simulink model "EcoSIM3_P2_C2"  (R2014b)
settings: Solver=ode1  SolverMode=SingleTasking  StartTime=0.0  StopTime=inf  FixedStep=0.01  RelTol=1e-3
PostLoadFcn:
  | %, if any(exist('dsrtsu_mdlpostloadfcn', 'file') == [2, 3, 6]), try dsrtsu_mdlpostloadfcn('Execute', bdroot); catch fprintf('Error in PostLoadFcn (dsrtsu_mdlpostloadfcn) for model "%s":\n %s\n', bdroot, lasterr); end, end,
InitFcn:
  | tic
  | %Startup_EcoSIM
values from neighbouring files (symbols this model uses):
  EngPwr = [0 5	10	15	20	25	30	35	40	45	50	55	60	65	70	75	80	85	90	95	100	105	110	115]    [Series_Maps.m]
  EngSpd = [0 477.4645 954.929 1909.858 2864.787 3819.716 4774.645 5729.574 6684.503]    [Series_Maps.m]
  EngTrq = [0	0	0	0	0	0	0	0	0	0	0	0	0	0	0	0	0	0	0	0	0	0	0	0 ... (first row only)    [Series_Maps.m]
  Power = [0 5 10 15 20 25 30]    [Series_Maps.m]
  Torque = [-50,-40,-30,-25,-20,-15,-10,-8,-6,-4,-2,0]    [Series_Maps.m]
undefined symbols (not defined in the file or in its folder): canChannel, Controls, DriveCycles, Driver, EM_EFF_MAP, EM_PwrLoss_MAP, Glbl, Plants, Veh_Dynamics
libraries: canmsglib x100, canlib x87, fl_lib x78, simulink x59, nesl_utility x40, sdl_lib x17, dspsigops x5, dspswit3 x3, dspstat3 x2, commnoisgen2 x1, dspfdesign x1
(part 1 of 15)
settings Model: DSRTSU_INTERNAL_RTI_VER=450  DSRTSU_INTERNAL_RTI_TYPE=rti1006  RTICANMMDATA=struct('GeneralSetupData',struct('modelroot','C:\Users\EcoCAR_HIL\Documents\Khanna\EcoSIM3_P1_0_PHEV_dynamic_RTI','generalsettings',struct('filesettings',struct('destfolder',struct('Name','RTICANMM_FILES','Check',1),'buildfolder',struct('Name','.','Check',1),'AbsDestfolder',struct('Name','C:\Users\EcoCAR_HIL\Documents\Khanna\EcoSIM3_P1_0_PHEV_dynamic_RTI\RTICANMM_FILES'),'AbsBuildfolder',struct('Name','C:\Users\EcoCAR_HIL\Documents\Khanna\EcoSIM3_P1_0_PHEV_dynamic_RTI'))),'options',struct('addpaths',1,'rmpaths',1,'addtrcexclusion',logical(1),'cannavigator',struct('checkmonitoring',0),'show_usrtrc',0,'use_usrtrc',0),'advanced',struct('options',[1 1 1 1 1 1 1 1 1 1 1 1 1 1 1 1 1 1 1 1 1 1 1 1 1 1 1 1 1 1 1 1 1 1 1 1 1 1 1 1 1 1 1 1 1 1 1 1 1 1 1 1 1 1 1 1 1 1 1 1 1 1 1 1 1 1 1 1 1 1 1 1 1 1 1 1 1 1 1 1 1 1 1 1 1 1 1 1 1 1 1 1 1 1 1 1 1 1 1 1]),'MPSetup',{{}},'modelname','EcoSIM3_P1_0_PHEV_2014b_with_inertia','block','EcoSIM3_P1_0_PHEV_2014b_with_inertia'))  DSRTSU_INTERNAL_RTIFPGA=40  Creator=Arjun  LastModifiedBy=EcoCAR_HIL
settings ConfigSet: Description=This configuration is meant for HIL simulations. During HIL simulations, the model should use dSPACE's rti1006 to generate code.
settings DataIOCC: InspectSignalLogs=on
settings OptimizationCC: BlockReduction=off
settings DebuggingCC: UnderspecifiedInitializationDetection=Classic  MergeDetectMultiDrivingBlocksExec=none  MultiTaskCondExecSysMsg=warning
settings HardwareCC: ProdIntDivRoundTo=Zero  ProdEndianess=LittleEndian  ProdHWDeviceType=Generic->Custom  TargetIntDivRoundTo=Zero  TargetEndianess=LittleEndian  TargetHWDeviceType=Generic->Custom
settings RTWCC: SystemTargetFile=rti1006.tlc  MakeCommand=make_rti  TemplateMakefile=rti1006.tmf  Description=dSPACE DS1006 Hardware Platform  ProcessScript=rti1006_make_rtw_hook
settings STFCustomTargetCC: ParMdlRefBuildCompliant=on  GeneratePreprocessorConditionals=Disable all  SystemTargetFile=rti1006.tlc
settings GRTTargetCC: CompOptLevelCompliant=off  ConcurrentExecutionCompliant=off  CombineOutputUpdateFcns=off  MatFileLogging=off  CPPClassGenCompliant=off  GRTInterface=on  ExtModeMexFile=noextcomm
settings SimscapeCC: SelectedTab=Simscape

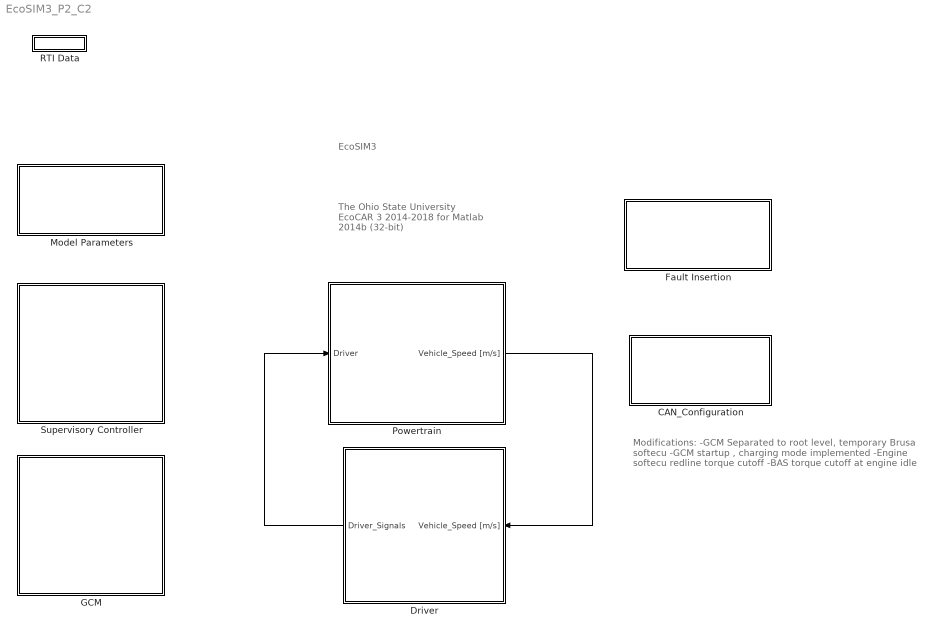
== system EcoSIM3_P2_C2 ==
  note: Modifications:
      | -GCM Separated to root level, temporary Brusa softecu
      | -GCM startup , charging mode implemented
      | -Engine softecu redline torque cutoff
      | -BAS torque cutoff at engine idle
  note: The Ohio State University
      | EcoCAR 3 2014-2018
      | for Matlab 2014b (32-bit)
  note: EcoSIM3
  CAN_Configuration : Subsystem  Variant=on  VariantControl=Sim_type == 1
  Driver : Subsystem
      mask Display: image(imread('images/BRUTUS.png'))
  Fault Insertion : Subsystem
  GCM : Subsystem  SystemSampleTime=0.001  VariantControl=Variant1
      settings: MinAlgLoopOccurrences=on
      mask Display: image(imread('images/GCM.jpg'))
  Model Parameters : Subsystem  mask{DRIV_cycle=US06 - City portion, Grade=0, Init_SOC=50}
      mask prompts: DRIV_cycle "Drive Cycle"; Grade "Grade [%]"; Init_SOC "Initial SOC [%]"
      mask help: Model Parameters Available for Modification
      mask TypeOptions DRIV_cycle: FUDS | FHDS | US06 | UDDS - 505 portion | US06 - City portion | US06 - Highway portion | Gradeability Test | Acceleration Test | Demo Cycle
      mask Display: disp('Simulation\nParameters')
  Powertrain : Subsystem
      mask Display: image(imread('images/OSU_EC3_Powertrain.png'))
  RTI Data : Subsystem  Tag=struct('RTIDataServer',struct('RTIDataServerVs','2','RTIModelDescription','struct(''main'',''EcoSIM3_P2_C2'',''sub'','''',''isMp'',0)'))  LoadFcn="if exist('rtidc'), try,  rtidc('DataHostBlockClbLoad', gcbh); catch, disp(['Warning: ''LoadFcn'' for RTI Data block failed: ' lasterr]); end, end,"  mask(RTI_DATA_HOST){}
      mask help:
      | RTI Data Block.
      | This block is used by RTI to store internal model-dependent data.
      | Please keep this block on the root level of the model. Deleting this block will result in data loss.
      |
      | NEVER DELETE OR COPY THIS BLOCK!
      settings: CopyFcn="if exist('rtidc'), try,  rtidc('DataHostBlockClbCopy', gcbh); catch, disp(['Warning: ''CopyFcn'' for RTI Data block failed: ' lasterr]); end, end,"  DeleteFcn="if exist('rtidc'), try,  rtidc('DataHostBlockClbDelete', gcbh); catch, disp(['Warning: ''DeleteFcn'' for RTI Data block failed: ' lasterr]); end, end,"  ModelCloseFcn="if exist('rtidc'), try,  rtidc('DataHostBlockClbModelClose', gcbh); catch, disp(['Warning: ''ModelCloseFcn'' for RTI Data block failed: ' lasterr]); end, end,"  PreSaveFcn="if exist('rtidc'), try,  rtidc('DataHostBlockClbPreSave', gcbh); catch, disp(['Warning: ''PreSaveFcn'' for RTI Data block failed: ' lasterr]); end, end,"  PostSaveFcn="if exist('rtidc'), try,  rtidc('DataHostBlockClbPostSave', gcbh); catch, disp(['Warning: ''PostSaveFcn'' for RTI Data block failed: ' lasterr]); end, end,"  NameChangeFcn="if exist('rtidc'), try,  rtidc('DataHostBlockClbNameChange', gcbh); catch, disp(['Warning: ''NameChangeFcn'' for RTI Data block failed: ' lasterr]); end, end,"
      mask Help:
      | RTI Data Block.
      | This block is used by RTI to store internal model-dependent data.
      | Please keep this block on the root level of the model. Deleting this block will result in data loss.
      | 
      | NEVER DELETE OR COPY THIS BLOCK!
      mask Display:
      | text(0.5, 0.5, 'RTI Data', 'HorizontalAlignment', 'center');
      | plot([1 0]);
  Supervisory Controller : Subsystem  SystemSampleTime=0.001  VariantControl=Variant1
      settings: MinAlgLoopOccurrences=on
      mask Display: image(imread('images/super.jpg'))
  wires:
  Powertrain/1(Vehicle_Speed [m/s]) -> Driver/1(Vehicle_Speed [m/s])
  Driver/1(Driver_Signals) -> Powertrain/1(Driver)

== system EcoSIM3_P2_C2/CAN_Configuration ==
  From_Goto : Subsystem  VariantControl=Sim_type == 1
  MIL_SIL_Kvaser : Subsystem  VariantControl=Sim_type == 3
  MIL_SIL_Vector : Subsystem  VariantControl=Sim_type == 2

== system EcoSIM3_P2_C2/Driver ==
  note: Driver
  Vehicle_Speed [m/s] : Inport
  APP : Subsystem
  Bus Creator : BusCreator  Inputs=5
  Bus Selector : BusSelector  OutputSignals=Velocity_Profile_m_per_s
  Bus Selector1 : BusSelector  OutputSignals=Vehicle_Speed_meter_per_s
  Drive_Mode : Constant
  GM_Transmit : Subsystem
  PI Controller : Subsystem
  PRNDL : Constant  Commented=on
  PRNDL_Input : Step  Time=1.8  Before=1  After=4  SampleTime=0
  Startup Dummy : Subsystem
  Driver_Signals : Outport
  wires:
  Bus Selector/1 -> PI Controller/1(Velocity_Profile [m/s])  "<Velocity_Profile_m_per_s>"
  PI Controller/1(Alpha [%]) -> APP/1(Pos_AccPedal[%])
  [Simulation_Parameters] -> Bus Selector/1
  PRNDL_Input/1 -> Startup Dummy/1(PRNDL), Bus Creator/2  "PRNDL"
  PI Controller/2(Beta [%]) -> Startup Dummy/2(Beta)
  Vehicle_Speed [m/s]/1 -> GM_Transmit/3(CAN2), Bus Selector1/1
  Bus Selector1/1 -> PI Controller/2(Vehicle_Speed [m/s]), Startup Dummy/3(VehSpeed)  "<Vehicle_Speed_meter_per_s>"
  Drive_Mode/1 -> Bus Creator/1  "Drive_Mode"
  APP/1(Accel_Low[V]) -> Bus Creator/3
  APP/2(Accel_High[V]) -> Bus Creator/4
  Startup Dummy/1(KeyState) -> Bus Creator/5
  GM_Transmit/1(Driver_Signals) -> Driver_Signals/1
  Bus Creator/1 -> GM_Transmit/1(Electrical)
  Startup Dummy/2(Vehicle Out) -> GM_Transmit/2(CAN1)

== system EcoSIM3_P2_C2/Fault Insertion ==
  EM_Inverter_Triggers : Subsystem
  ESS Triggers : Subsystem

== system EcoSIM3_P2_C2/GCM ==
  note: Do we have to use the supervisory wakeup signal in MIL?
      | We could put the RTI DIG block in the GCM built model to
      | power up the supervisory
  Bus Creator1 : BusCreator  Inputs=1
  Bus Creator2 : BusCreator  Inputs=2
  GCM_IO : Subsystem  Variant=on
  ProcessMode : Subsystem
  tag scope: GCM_To_CAN=global
  wires:
  [GCM_from_CAN] -> ProcessMode/1(In1)
  ProcessMode/1(ChargeModeRequest) -> Bus Creator1/1
  Bus Creator1/1 -> Bus Creator2/1  "GCM_CAN_Out"
  Bus Creator2/1 -> [GCM_To_CAN]  "GCM_Transmit"
  ProcessMode/2(RelaySignals) -> Bus Creator2/2  "GCM_Electrical_Out"

== system EcoSIM3_P2_C2/Model Parameters ==
  Bus Creator : BusCreator  Inputs=2
  Clock : Clock
  Cycle Length : Subsystem
  Drive Cycle : Constant  Value=DRIV_cycle
  Drive Cycle Selection : Subsystem
  Initial_SOC : Constant  Value=Init_SOC
  Relational Operator2 : RelationalOperator  InputSameDT=on
  Stop Simulation : Stop
  tag scope: Simulation_Parameters=global
  wires:
  Bus Creator/1 -> [Simulation_Parameters]  "Simulation_Parameters"
  Relational Operator2/1 -> Stop Simulation/1
  Clock/1 -> Relational Operator2/1  "sim_time"
  Initial_SOC/1 -> Bus Creator/2  "Init_SOC_percent"
  Drive Cycle Selection/1(Cycle Velocity) -> Bus Creator/1
  Cycle Length/1(Cycle Time) -> Relational Operator2/2
  Drive Cycle/1 -> Drive Cycle Selection/1(Drive Cyc Selection), Cycle Length/1(Drive Cyc Selection)

== system EcoSIM3_P2_C2/Powertrain ==
  note: Powertrain
  Driver : Inport
  Accessories : Subsystem
      mask Display: image(imread('images/acc.jpg'))
  BAS Motor : Subsystem
      mask Display: image(imread('images/BAS.png'))
  Belt Coupler : Subsystem
      mask Display: image(imread('images/'))
  Bus Selector : BusSelector  OutputSignals=GMLAN_CAN_Out.PPEI_Brake_Apply_Status.BrkPdlPos
  Charger : Subsystem
      mask Display: image(imread('images/charger.jpg'))
  Charger Plug In : Constant  Value=0
  Clutch_Transmission2 : Subsystem
  "Electric Motor " : Subsystem
      mask Display: image(imread('images/EM.png'))
  Electrical Storage System : Subsystem
      mask Display: image(imread('images/ESS.png'))
  Engine : Subsystem
      mask Display: image(imread('images/Engine.png'))
  Fuel Tank : Subsystem
      mask Display: image(imread('images/Fuel_Tank.png'))
  Mechanical Coupler : Subsystem
      mask Display: image(imread('images/PTU.png'))
  Soft_ECUs_IO : Subsystem  Variant=on
  Vehicle Dynamics : Subsystem
      mask Display: image(imread('images/2016camaro.png'))
  Vehicle_Speed [m/s] : Outport
  tag scope: GM_Transmit=global
  wires:
  Accessories/1(Accessories_Power_In_W) -> Electrical Storage System/2(Accessories_Power_In [W])
  "Electric Motor "/1(To_Battery) -> Electrical Storage System/3(EM_Power_In [W])
  BAS Motor/1(BAS_Power_in [W]) -> Electrical Storage System/4(BAS_Power_In [W])
  Engine/1(Fuel_Consumption) -> Fuel Tank/1(ICE_m_f_dot [kg/s])
  Vehicle Dynamics/1(Vehicle_Speed [m/s]) -> Vehicle_Speed [m/s]/1
  Bus Selector/1 -> Vehicle Dynamics/1(Beta)  "<BrkPdlPos>"
  Driver/1 -> [GM_Transmit], Bus Selector/1
  Charger Plug In/1 -> Charger/1(ACSupply)
  Charger/1(Charger_Power_W) -> Electrical Storage System/1(Charger_Power_In [W])
  connections:
  Engine/RConn1 -- Belt Coupler/LConn2
  Mechanical Coupler/RConn1 -- Vehicle Dynamics/LConn1
  "Electric Motor "/RConn1 -- Mechanical Coupler/LConn1
  Mechanical Coupler/LConn2 -- Clutch_Transmission2/RConn1
  Belt Coupler/RConn1 -- Clutch_Transmission2/LConn1
  BAS Motor/RConn1 -- Belt Coupler/LConn1

== system EcoSIM3_P2_C2/RTI Data ==
  RTI Data Store : Subsystem  Tag=struct('private',struct('version',struct('dsVer',uint32(2)),'access',struct('modified',['23-Sep-2016 18:03:14'],'type','Model','isPerm',1)),'public',struct('main',struct('data',[]),'sub',struct('name','','data',[])))  mask(RTI_DATA_STORE){}
      mask help:
      | RTI Data Store Block. This block is used by RTI to store internal model dependent data. Deleting this block will result in data loss.
      |
      | NEVER DELETE, COPY, OR MODIFY THIS BLOCK!
      mask Help:
      | RTI Data Store Block. This block is used by RTI to store internal model dependent data. Deleting this block will result in data loss.
      | 
      | NEVER DELETE, COPY, OR MODIFY THIS BLOCK!
      mask Display: text(0.5, 0.5, ' ', 'HorizontalAlignment', 'center');

== system EcoSIM3_P2_C2/Supervisory Controller ==
  Bus Creator1 : BusCreator  Inputs=2
  Bus Selector : BusSelector  OutputSignals=Vehicle_Ready
  Driver Requested Torque : Subsystem
  Functional Safety1 : Subsystem  Commented=on
  Input Conditioning : Subsystem
  Memory1 : Memory
  Mode Operation : Subsystem
  "Mode Selection " : Subsystem
  Outout Conditioning : Subsystem
  PRNDL : Subsystem
  Simple Fault Detection : Subsystem
  Supervisory_IO : Subsystem  Variant=on
  tag scope: To_Vehicle=global
  wires:
  [From_Vehicle] -> Input Conditioning/1(Raw Signals), Simple Fault Detection/1(In1)
  "Mode Selection "/1(Mode Transmit) -> Bus Creator1/2  "Mode"
  Driver Requested Torque/1(Driver Torque Request) -> Bus Creator1/1
  Memory1/1 -> "Mode Selection "/3(Startup)
  Simple Fault Detection/1("Fault Code ") -> "Mode Selection "/2("Fault_Code ")
  Bus Creator1/1 -> Mode Operation/1(Supervisory)
  Input Conditioning/1(Conditioned Signals) -> PRNDL/2("From CAN "), Mode Operation/2(From CAN), "Mode Selection "/1(CAN IN), Driver Requested Torque/1(CAN IN)
  PRNDL/1("Total Torque ") -> Outout Conditioning/1(In1)
  Mode Operation/1(Component Torque Request) -> PRNDL/1(Controller Inputs), Bus Selector/1
  Bus Selector/1 -> Memory1/1  "<Vehicle_Ready>"
  Outout Conditioning/1(Out1) -> [To_Vehicle]

== system EcoSIM3_P2_C2/CAN_Configuration/From_Goto ==
  Ground : Ground
  Terminator : Terminator
  wires:
  Ground/1 -> Terminator/1

== system EcoSIM3_P2_C2/CAN_Configuration/MIL_SIL_Kvaser ==
  CAN Configuration : canlib/CAN Configuration  BlockHandle=18.0005  DeviceMenu=Kvaser Virtual 1 (Channel 1)  Device=Kvaser Virtual 1 (Channel 1)  ObjConstructor=canChannel('Kvaser', 'Virtual 1', 1)  BusSpeed=500000  EnableBitParameters=off  SJW=1  TSEG1=4  TSEG2=3  NSamples=1  AckMode=Normal
  CAN Configuration1 : canlib/CAN Configuration  BlockHandle=19.0005  DeviceMenu=Kvaser Virtual 1 (Channel 2)  Device=Kvaser Virtual 1 (Channel 2)  ObjConstructor=canChannel('Kvaser', 'Virtual 1', 2)  BusSpeed=500000  EnableBitParameters=off  SJW=1  TSEG1=4  TSEG2=3  NSamples=1  AckMode=Normal

== system EcoSIM3_P2_C2/CAN_Configuration/MIL_SIL_Vector ==
  CAN Configuration : canlib/CAN Configuration  BlockHandle=2713.0127  DeviceMenu=Vector Virtual 1 (Channel 1)  Device=Vector Virtual 1 (Channel 1)  ObjConstructor=canChannel('Vector', 'Virtual 1', 1)  BusSpeed=500000  EnableBitParameters=off  SJW=1  TSEG1=4  TSEG2=3  NSamples=1  AckMode=Normal
  CAN Configuration1 : canlib/CAN Configuration  BlockHandle=2789.0128  DeviceMenu=Vector Virtual 1 (Channel 2)  Device=Vector Virtual 1 (Channel 2)  ObjConstructor=canChannel('Vector', 'Virtual 1', 2)  BusSpeed=500000  EnableBitParameters=off  SJW=1  TSEG1=4  TSEG2=3  NSamples=1  AckMode=Normal

== system EcoSIM3_P2_C2/Driver/APP ==
  Pos_AccPedal[%] : Inport
  Add : Sum  Commented=on
  Constant : Constant  Value=.4
  Constant1 : Constant  Value=.8
  Constant2 : Constant  Commented=on  Value=.4
  Constant3 : Constant  Commented=on  Value=.8
  Constant4 : Constant  Commented=on  Value=40
  Constant5 : Constant  Commented=on  Value=.4
  Constant6 : Constant  Commented=on  Value=.8
  Display : Display  Commented=on
  Gain_APM1 : Gain  Gain=0.0021
  Offset_APM1 : Constant  Value=0.009
  Output Scaling1 : Gain  Gain=1/50
  Output Scaling2 : Gain  Gain=1/25
  Output Scaling3 : Gain  Commented=on  Gain=1/50
  Output Scaling4 : Gain  Commented=on  Gain=1/25
  Output Scaling5 : Gain  Commented=on  Gain=50
  Output Scaling6 : Gain  Commented=on  Gain=25
  Output Scaling7 : Gain  Commented=on  Gain=0.5
  Sum : Sum  Inputs=++|
  Sum1 : Sum  Inputs=|++
  Sum2 : Sum  Commented=on  Inputs=++|
  Sum3 : Sum  Commented=on  Inputs=|++
  Sum4 : Sum  Commented=on  Inputs=-+|
  Sum5 : Sum  Commented=on  Inputs=|+-
  Sum6 : Sum  Inputs=++|
  Accel_Low[V] : Outport
  Accel_High[V] : Outport  Port=2
  wires:
  Constant/1 -> Sum/1
  Sum/1 -> Accel_Low[V]/1  "Alpha_Low"
  Output Scaling1/1 -> Sum/2
  Pos_AccPedal[%]/1 -> Output Scaling2/1, Output Scaling1/1
  Constant1/1 -> Sum1/2
  Output Scaling2/1 -> Sum1/1
  Sum1/1 -> Accel_High[V]/1  "Alpha_High"
  Constant2/1 -> Sum2/1
  Sum2/1 -> Sum4/2  "Alpha_Low"
  Output Scaling3/1 -> Sum2/2
  Constant4/1 -> Output Scaling4/1, Output Scaling3/1
  Constant3/1 -> Sum3/2
  Output Scaling4/1 -> Sum3/1
  Sum3/1 -> Sum5/1  "Alpha_High"
  Constant5/1 -> Sum4/1
  Constant6/1 -> Sum5/2
  Sum4/1 -> Output Scaling5/1
  Sum5/1 -> Output Scaling6/1
  Output Scaling5/1 -> Add/1
  Output Scaling6/1 -> Add/2
  Add/1 -> Output Scaling7/1
  Output Scaling7/1 -> Display/1
  Sum6/1 -> ?  "Alpha_Low"
  ? -> Gain_APM1/1
  Gain_APM1/1 -> Sum6/2
  Offset_APM1/1 -> Sum6/1

== system EcoSIM3_P2_C2/Driver/GM_Transmit ==
  Electrical : Inport
  CAN1 : Inport  Port=2
  CAN2 : Inport  Port=3
  Bus Creator : BusCreator  Inputs=2
  Bus Creator1 : BusCreator  Inputs=5
  Bus Creator2 : BusCreator  Inputs=5
  Bus Creator3 : BusCreator  Inputs=2
  Bus Creator4 : BusCreator  Inputs=2
  Bus Creator5 : BusCreator  Inputs=1
  Bus Creator6 : BusCreator  Inputs=1
  Bus Creator7 : BusCreator  Inputs=1
  Bus Selector : BusSelector  OutputSignals=Drive_Mode,PRNDL,Alpha_Low,Alpha_High,Key_State
  Bus Selector1 : BusSelector  OutputSignals=SysPwrMd,BrkPdlPos,Vehicle_Speed_meter_per_s
  Bus Selector2 : BusSelector  OutputSignals=Rear_Right_Tire_Angle,Rear_Left_Tire_Angle,Front_Right_Tire_Angle,Front_Left_Tire_Angle
  Display : Display
  Gain : Gain  Gain=3.6
  Gain1 : Gain
  WheelTickLD : Subsystem
  WheelTickLND : Subsystem
  WheelTickRD : Subsystem
  WheelTickRND : Subsystem
  Driver_Signals : Outport
  wires:
  Bus Creator4/1 -> Bus Creator2/5  "PPEI_NonDrivn_Whl_Rotationl_Stat"
  CAN1/1 -> Bus Selector1/1
  Bus Creator1/1 -> Bus Creator/1  "GM_Electrical_Out"
  Bus Creator3/1 -> Bus Creator2/4  "PPEI_Driven_Whl_Rotational_Stat"
  Electrical/1 -> Bus Selector/1
  Bus Creator/1 -> Driver_Signals/1  "GM_Transmit"
  Bus Creator2/1 -> Bus Creator/2  "GMLAN_CAN_Out"
  Bus Selector/1 -> Bus Creator1/1  "<Drive_Mode>"
  Bus Selector/2 -> Bus Creator1/2  "<PRNDL>"
  Bus Selector/3 -> Bus Creator1/3  "<Alpha_Low>"
  Bus Selector/4 -> Bus Creator1/4  "<Alpha_High>"
  Bus Selector/5 -> Bus Creator1/5  "<Key_State>"
  Bus Creator5/1 -> Bus Creator2/2  "PPEI_Brake_Apply_Status"
  Bus Selector1/1 -> Gain1/1  "<SysPwrMd>"
  Bus Creator6/1 -> Bus Creator2/1  "PPEI_Platform_General_Status"
  Bus Selector1/3 -> Gain/1  "<Vehicle_Speed_meter_per_s>"
  Gain/1 -> Bus Creator7/1  "VehSpdAvgDrvn"
  Bus Creator7/1 -> Bus Creator2/3  "PPEI_Vehicle_Speed_and_Distance"
  CAN2/1 -> Bus Selector2/1
  Bus Selector2/4 -> WheelTickLND/1(In1)  "<Front_Left_Tire_Angle>"
  Bus Selector2/2 -> WheelTickLD/1(In1)  "<Rear_Left_Tire_Angle>"
  Bus Selector2/3 -> WheelTickRND/1(In1)  "<Front_Right_Tire_Angle>"
  Bus Selector2/1 -> WheelTickRD/1(In1)  "<Rear_Right_Tire_Angle>"
  Bus Selector1/2 -> Bus Creator5/1  "<BrkPdlPos>"
  Gain1/1 -> Display/1, Bus Creator6/1  "SysPwrMd"
  WheelTickRD/1(Out1) -> Bus Creator3/1
  WheelTickLD/1(Out1) -> Bus Creator3/2
  WheelTickRND/1(Out1) -> Bus Creator4/1
  WheelTickLND/1(Out1) -> Bus Creator4/2

== system EcoSIM3_P2_C2/Driver/PI Controller ==
  note: The accelerator override is used to press the ac pedal to check ac pedal startup requirement.
  Velocity_Profile [m/s] : Inport
  Vehicle_Speed [m/s] : Inport  Port=2
  Ac Pedal Override : Constant  Value=0
  Brake_Override : Constant  Commented=on  Value=0
  Compare To Zero1 : simulink/Logic and Bit Operations/Compare To Zero  relop===  OutDataTypeStr=boolean  ZeroCross=off
  Delay : Subsystem
  I : Constant  Value=Driver.I
  Integrator1 : Integrator  ExternalReset=level
  P : Constant  Value=Driver.P
  Percent_alpha : Constant  Value=10
  Product3 : Product  RndMeth=Zero
  Product4 : Product  RndMeth=Zero
  Saturation (-1 to 0)1 : Saturate  UpperLimit=0  LowerLimit=-100
  Saturation (0 to 1)1 : Saturate  UpperLimit=100  LowerLimit=0
  Step : Step  Time=5  After=100  SampleTime=0
  Sum3 : Sum  Inputs=|-+  SaturateOnIntegerOverflow=on  InputSameDT=on  OutDataTypeStr=Inherit: Same as first input
  Sum4 : Sum  SaturateOnIntegerOverflow=on  InputSameDT=on  OutDataTypeStr=Inherit: Same as first input
  Sum5 : Sum  Inputs=|+-  SaturateOnIntegerOverflow=on  InputSameDT=on  OutDataTypeStr=Inherit: Same as first input
  Switch : Switch  Criteria=u2 > Threshold  Threshold=0.5
  gain1 : Gain  Gain=-1  SaturateOnIntegerOverflow=on  OutDataTypeStr=Inherit: Same as input  ParamDataTypeStr=Inherit: Same as input
  Alpha [%] : Outport
  Beta [%] : Outport  Port=2
  wires:
  Saturation (-1 to 0)1/1 -> gain1/1
  Sum4/1 -> Saturation (0 to 1)1/1, Saturation (-1 to 0)1/1
  Vehicle_Speed [m/s]/1 -> Sum3/1, Compare To Zero1/1, Sum5/2
  Product4/1 -> Sum4/1
  Product3/1 -> Sum4/2
  Compare To Zero1/1 -> Integrator1/2
  Integrator1/1 -> Product3/1
  Velocity_Profile [m/s]/1 -> Sum5/1, Delay/1(Velocity_Profile [m/s])
  Sum5/1 -> Product4/2
  Switch/1 -> Alpha [%]/1  "Alpha_percentage"
  Delay/1(Pre_Velocity_Profile [m/s]) -> Sum3/2
  Sum3/1 -> Integrator1/1
  I/1 -> Product3/2
  P/1 -> Product4/1
  gain1/1 -> Beta [%]/1  "Beta_percentage"
  Ac Pedal Override/1 -> Switch/2
  Step/1 -> Switch/1
  Saturation (0 to 1)1/1 -> Switch/3

== system EcoSIM3_P2_C2/Driver/Startup Dummy ==
  note: Key_Sw is the electrical signal to wake the GCM. It is triggered by either
      | the push button or plugging the Brusa in.
  note: VehStart is a processed signal to emulate SysPwrMd in GMLAN
  PRNDL : Inport
  Beta : Inport  Port=2
  VehSpeed : Inport  Port=3
  Bus Creator : BusCreator  Inputs=3
  Bus Selector : BusSelector  OutputSignals=Brusa_Electrical_Out.GCM_Wakeup_charge
  Chart : Stateflow chart  TreatAsAtomicUnit=on
  Logical Operator : Logic  Operator=OR  AllPortsSameDT=off  OutDataTypeStr=boolean
  Start Button : Step  Before=1  After=0  SampleTime=0
  Terminator : Terminator
  Vehicle Start : Subsystem
  KeyState : Outport
  Vehicle Out : Outport  Port=2
  wires:
  Start Button/1 -> Vehicle Start/2(Key Pos), Chart/1(input)  "Key_State"
  Logical Operator/1 -> Terminator/1  "Key_Sw"
  [Brusa_SoftECU_Transmit] -> Bus Selector/1
  Vehicle Start/2(SysPwrMd) -> Bus Creator/1  "SysPwrMd"
  Beta/1 -> Vehicle Start/3(Brake_Position)
  Vehicle Start/3(Brake Position) -> Bus Creator/2
  Bus Creator/1 -> Vehicle Out/1  "CAN"
  VehSpeed/1 -> Bus Creator/3
  Bus Selector/1 -> Logical Operator/2  "<GCM_Wakeup_charge>"
  Vehicle Start/1(Key State) -> KeyState/1
  Chart/1(output) -> Logical Operator/1
  PRNDL/1 -> Vehicle Start/1(PRNDL)

== system EcoSIM3_P2_C2/Fault Insertion/EM_Inverter_Triggers ==
  Bus Creator{,1..2,4} (4 alike) : BusCreator  Inputs=2
  EM_Faulty_Temperature : Constant  Value=0
  EM_Inverter_Faulty_Temperature : Constant  Value=0
  EM_torque_cmd_rigger : Step  Time=18  After=0  SampleTime=0
  EM_torque_cmd_value : Constant  Value=0
  Step : Step  Time=18  After=0  SampleTime=0
  Trigger : Step  Time=18  After=0  SampleTime=0
  Trigger1 : Step  Time=18  After=0  SampleTime=0
  vsm_state_trigger : Step  Time=18  After=0  SampleTime=0
  vsm_state_value : Constant  Value=0
  tag scope: EM_Inverter_Over_temperature_Trigger=global, EM_OverTorque_Trigger=global, EM_Over_temperature_Trigger=global, EM_Torque_Cmd_Trigger=global, VSM_State_Trigger=global
  wires:
  Bus Creator4/1 -> [VSM_State_Trigger]  "vsm_state_fault"
  vsm_state_trigger/1 -> Bus Creator4/1  "vsm_state_trigger"
  vsm_state_value/1 -> Bus Creator4/2  "vsm_state_value"
  Trigger/1 -> Bus Creator/1  "EM_OverTemp_Trigger"
  Step/1 -> [EM_OverTorque_Trigger]  "EM_OverTorque_Fault_trigger"
  Bus Creator/1 -> [EM_Over_temperature_Trigger]  "EM_Over_Temperature_Fault"
  EM_Faulty_Temperature/1 -> Bus Creator/2  "Temp_deg_C"
  Bus Creator1/1 -> [EM_Inverter_Over_temperature_Trigger]  "EM_Inverter_Over_Temperature_Fault"
  EM_Inverter_Faulty_Temperature/1 -> Bus Creator1/2  "Temp_deg_C"
  Trigger1/1 -> Bus Creator1/1  "EM_Inverter_OverTemp_Trigger"
  Bus Creator2/1 -> [EM_Torque_Cmd_Trigger]  "vsm_state_fault"
  EM_torque_cmd_rigger/1 -> Bus Creator2/1  "EM_torque_cmd_trigger"
  EM_torque_cmd_value/1 -> Bus Creator2/2  "EM_torque_cmd_value"

== system EcoSIM3_P2_C2/Fault Insertion/ESS Triggers ==
  Bus Creator2 : BusCreator  Inputs=2
  Bus Creator3 : BusCreator  Inputs=2
  Chart : Stateflow chart  Commented=on  TreatAsAtomicUnit=on
  ESS_Faulty_Temperature : Constant  Value=0
  Trigger2 : Step  Time=18  After=0  SampleTime=0
  bcm_alarm_trigger : Step  Time=18  After=0  SampleTime=0
  bcm_alarm_type : Constant  Value=0
  tag scope: BCM_Alarm_Trigger=global, ESS_Over_temperature_Trigger=global
  wires:
  Trigger2/1 -> Bus Creator2/1  "ESS_OverTemp_Trigger"
  Bus Creator2/1 -> [ESS_Over_temperature_Trigger]  "ESS_Over_Temperature_Fault"
  ESS_Faulty_Temperature/1 -> Bus Creator2/2  "Temp_deg_C"
  Bus Creator3/1 -> [BCM_Alarm_Trigger]  "bcm_alarm_fault"
  bcm_alarm_trigger/1 -> Bus Creator3/1  "bcm_alarm_trigger"
  bcm_alarm_type/1 -> Bus Creator3/2  "bcm_alarm_type"
  ? -> Chart/1(in)  "ESS_OverTemp_Trigger"

== system EcoSIM3_P2_C2/GCM/GCM_IO ==
  note: 1) Add Subsystem or Model blocks as valid variant choices.
      | 2) You cannot connect blocks at this level. At simulation, connectivity is automatically
      | determined, based on the active variant and port name matching.
  From_Goto : Subsystem  VariantControl=Sim_type == 1
  VNT Kvaser : Subsystem  VariantControl=Sim_type == 3
  VNT Vector : Subsystem  VariantControl=Sim_type == 2

== system EcoSIM3_P2_C2/GCM/ProcessMode ==
  note: SWREL12 is the relay signal to power up the remaining softECUs
  note: SWREL11 is the relay signal to power up the MABx, A123, and DCDC
  In1 : Inport
  Bus Creator : BusCreator  Inputs=2
  Bus Selector : BusSelector  OutputSignals=GM_Transmit.GM_Electrical_Out.Key_State,Brusa_Transmit.Brusa_Electrical_Out.GCM_Wakeup_charge
  Chart : Stateflow chart  TreatAsAtomicUnit=on
  ChargeModeRequest : Outport
  RelaySignals : Outport  Port=2
  wires:
  In1/1 -> Bus Selector/1
  Bus Creator/1 -> RelaySignals/1
  Chart/1(charge_mode_request) -> ChargeModeRequest/1
  Bus Selector/1 -> Chart/1(Key_State)  "<Key_State>"
  Bus Selector/2 -> Chart/2(GCM_Wakeup_charge)  "<GCM_Wakeup_charge>"
  Chart/2(Relay_Charge) -> Bus Creator/1  "Relay_Charge"
  Chart/3(Relay_Vehicle) -> Bus Creator/2  "Relay_Vehicle"

== system EcoSIM3_P2_C2/Model Parameters/Cycle Length ==
  Drive Cyc Selection : Inport
  Multiport Switch : MultiPortSwitch  Inputs=9
  Time : Constant  Value=length(DriveCycles.FUDS.t_cyc)
  Time1 : Constant  Value=length(DriveCycles.FHDS.t_cyc)
  Time2 : Constant  Value=length(DriveCycles.US06.t_cyc)
  Time3 : Constant  Value=length(DriveCycles.Cycle_505.t_cyc)
  Time4 : Constant  Value=length(DriveCycles.US06_City.t_cyc)
  Time5 : Constant  Value=length(DriveCycles.US06_Highway.t_cyc)
  Time6 : Constant  Value=length(DriveCycles.Gradeability.t_cyc)
  Time7 : Constant  Value=length(DriveCycles.Acceleration.t_cyc)
  Time8 : Constant  Value=100
  Cycle Time : Outport
  wires:
  Time/1 -> Multiport Switch/2
  Time1/1 -> Multiport Switch/3
  Time2/1 -> Multiport Switch/4
  Time3/1 -> Multiport Switch/5
  Time4/1 -> Multiport Switch/6
  Time5/1 -> Multiport Switch/7
  Time6/1 -> Multiport Switch/8
  Time7/1 -> Multiport Switch/9
  Drive Cyc Selection/1 -> Multiport Switch/1
  Multiport Switch/1 -> Cycle Time/1
  Time8/1 -> Multiport Switch/10

== system EcoSIM3_P2_C2/Model Parameters/Drive Cycle Selection ==
  note: Parameterize-
      | RampSlope
  Drive Cyc Selection : Inport
  505 : simulink/Sources/Repeating Sequence  rep_seq_t=DriveCycles.Cycle_505.t_cyc  rep_seq_y=DriveCycles.Cycle_505.v_cyc
  Acceleration : simulink/Sources/Repeating Sequence  rep_seq_t=DriveCycles.Acceleration.t_cyc  rep_seq_y=DriveCycles.Acceleration.v_cyc
  Demo Cycle : Subsystem
  FHDS : simulink/Sources/Repeating Sequence  rep_seq_t=DriveCycles.FHDS.t_cyc  rep_seq_y=DriveCycles.FHDS.v_cyc
  FUDS : simulink/Sources/Repeating Sequence  rep_seq_t=DriveCycles.FUDS.t_cyc  rep_seq_y=DriveCycles.FUDS.v_cyc
  Gradeability : simulink/Sources/Repeating Sequence  rep_seq_t=DriveCycles.Gradeability.t_cyc  rep_seq_y=DriveCycles.Gradeability.v_cyc
  Multiport Switch : MultiPortSwitch  Inputs=9
  US06 : simulink/Sources/Repeating Sequence  rep_seq_t=DriveCycles.US06.t_cyc  rep_seq_y=DriveCycles.US06.v_cyc
  US06_City : simulink/Sources/Repeating Sequence  rep_seq_t=DriveCycles.US06_City.t_cyc  rep_seq_y=DriveCycles.US06_City.v_cyc
  US06_Highway : simulink/Sources/Repeating Sequence  rep_seq_t=DriveCycles.US06_Highway.t_cyc  rep_seq_y=DriveCycles.US06_Highway.v_cyc
  Cycle Velocity : Outport
  wires:
  Multiport Switch/1 -> Cycle Velocity/1  "Velocity_Profile_m_per_s"
  FUDS/1 -> Multiport Switch/2
  FHDS/1 -> Multiport Switch/3
  US06/1 -> Multiport Switch/4
  505/1 -> Multiport Switch/5
  US06_City/1 -> Multiport Switch/6
  US06_Highway/1 -> Multiport Switch/7
  Gradeability/1 -> Multiport Switch/8
  Acceleration/1 -> Multiport Switch/9
  Drive Cyc Selection/1 -> Multiport Switch/1
  Demo Cycle/1(v) -> Multiport Switch/10

== system EcoSIM3_P2_C2/Powertrain/Accessories ==
  Add : Sum
  Bus Selector : BusSelector  OutputSignals=ESS_CAN_Out.BCM_Status.bcm_vbat
  Constant : Constant
  Constant1 : Constant  Value=12
  Constant2 : Constant  Value=28
  Constant3 : Constant  Value=30
  Constant4 : Constant  Value=4.41
  DCDC avg current_A : Constant  Value=1.7918
  HVAC : Subsystem
  Memory : Memory
  Parameters : Subsystem
  Product : Product
  Rate Transition1 : RateTransition
  The Corrupter : Subsystem
  Accessories_Power_In_W : Outport
  wires:
  Add/1 -> Rate Transition1/1  "Accessories_Power_In_W"
  Rate Transition1/1 -> Accessories_Power_In_W/1
  [ESS_SoftECU_Transmit] -> Bus Selector/1
  Bus Selector/1 -> Memory/1  "<bcm_vbat>"
  DCDC avg current_A/1 -> The Corrupter/1(Signal In)
  Product/1 -> Add/2
  Memory/1 -> HVAC/6(Voltage), Product/2
  HVAC/1(HVAC Pwr_W) -> Add/1
  Constant/1 -> HVAC/1(AC_Mode)
  Constant1/1 -> HVAC/2(AC_Press_bar)
  Constant2/1 -> HVAC/3(AC_Engagement_pressure)
  Constant3/1 -> HVAC/4(AC_max_pressure)
  Constant4/1 -> HVAC/5(Current)
  The Corrupter/1(Signal Out) -> Product/1  "APM_Current"
  Parameters/1(P) -> The Corrupter/2(Noise Parameters)

== system EcoSIM3_P2_C2/Powertrain/BAS Motor ==
  note: Power IN or OUT goes to battery????!!
  note: BAS
  " Compnent Model" : Subsystem
  BAS_Receive : Subsystem
  BAS_Transmit : Subsystem
  Soft ECU : Subsystem
  To_Plants : PMIOPort  Port=1  Side=Right
  BAS_Power_in [W] : Outport
  wires:
  " Compnent Model"/2(To_Battery) -> BAS_Power_in [W]/1
  " Compnent Model"/1(Sensor_Out) -> Soft ECU/2(Sensor_In)
  Soft ECU/2(Actuator_Cmds) -> " Compnent Model"/1(Actuator_Cmds)
  Soft ECU/1(CAN_Out) -> BAS_Transmit/1(To_ECUs)
  BAS_Receive/1(From_ECUs) -> Soft ECU/1(CAN_In)
  connections:
  To_Plants/RConn1 -- " Compnent Model"/RConn1

== system EcoSIM3_P2_C2/Powertrain/Belt Coupler ==
  note: to the BAS
  note: BELT COUPLER
  Belt Drive : sdl_lib/Couplings & Drives/Belt Drive  Commented=on  drive_type=1  belt_type=2  sheave_ang=30 deg  num_belts=8  linear_density=0.6 kg/m  stiffness=1e+4 N/m  damping=1000 N/(m/s)  tension=698 N  breakable=0  F_max=1e+5 N  r_pulley_A=1.1353 in  r_pulley_B=2.8028 in  b_pulley_A=0.001 N*m/(rad/s)  b_pulley_B=0.001 N*m/(rad/s)  model_inertia_A=1  model_inertia_B=1  pulley_inertia_A=0.00001 kg*m^2  pulley_inertia_B=0.00001 kg*m^2  initial_velocity_A=0 rad/s  initial_velocity_B=0 rad/s  mu=0.5  wrap_parameterization=1  d_centers=10.0894 in  phi_wrap_A=145 deg  phi_wrap_B=215 deg  v_thr=0.001 m/s
      settings: LogSimulationData=on
  Sensors : Subsystem
  Simple Gear : sdl_lib/Gears/Simple Gear  ratio=Plants.Belt.GR  rotation_direction=1  friction_model=1  T_noload=0.1 N*m  T_nom=5 N*m  efficiency_nom=0.8  efficiency=0.8  mu_visc=[ 0 0 ] N*m/(rad/s)  w_thr=0.01 rad/s
  BAS Output Shaft1 : PMIOPort  Tag=PMCPort  Port=1  Side=Left
  ICE Output Shaft : PMIOPort  Tag=PMCPort  Port=2  Side=Left
  To_Clutch : PMIOPort  Tag=PMCPort  Port=3  Side=Right
  connections:
  ICE Output Shaft/RConn1 -- Simple Gear/RConn1 -- Sensors/LConn1
  To_Clutch/RConn1 -- Sensors/RConn1
  Simple Gear/LConn1 -- BAS Output Shaft1/RConn1

== system EcoSIM3_P2_C2/Powertrain/Charger ==
  note: Charger
  ACSupply : Inport
  CAN_Revieve : Subsystem
  CAN_Transmit : Subsystem
  Plant : Subsystem
  Soft ECU : Subsystem
  Charger_Power_W : Outport
  wires:
  ACSupply/1 -> Soft ECU/2(AC)
  CAN_Revieve/1(From_ECUs) -> Soft ECU/1(FromESS)
  Soft ECU/1(ToECUs) -> CAN_Transmit/1(To_CAN)
  Soft ECU/2(Actuator_Cmds) -> Plant/1(FromSoftECU)
  Plant/1(To Plant) -> Charger_Power_W/1

== system EcoSIM3_P2_C2/Powertrain/Clutch_Transmission2 ==
  note: Clutch
  note: Transmission
  Bus Creator : BusCreator  Inputs=2
  Bus Creator1 : BusCreator  Inputs=2
  Bus Creator2 : BusCreator  Inputs=2
  CAN_Recieve : Subsystem
  CAN_Transmit : Subsystem
  CP1 SoftEcu : Subsystem  Commented=on
  Clutch_Plant : Subsystem
  GCM : Subsystem
  Mastershift Softecu : Subsystem  Commented=on
  Terminator : Terminator
  Trans_Plant : Subsystem
  Shaft : PMIOPort  Tag=PMCPort  Port=1  Side=Left
  Trans Output Shaft : PMIOPort  Port=2  Side=Right
  wires:
  Trans_Plant/1(Sensor_Out) -> Bus Creator/2
  Clutch_Plant/1(Clutch_Status) -> Bus Creator/1
  Bus Creator/1 -> Mastershift Softecu/3(Sensor_In), CP1 SoftEcu/2(Sensor_In)  "Sensor_Out"
  CAN_Recieve/1(From_CAN) -> Trans_Plant/1(Gear_Cmd), GCM/1(CAN_In)
  CP1 SoftEcu/1(To_GCM) -> Bus Creator1/1, Mastershift Softecu/2(Clutch_CAN_Out)
  CP1 SoftEcu/2(Actuator_Cmds) -> Clutch_Plant/1(Clutch_Engage)
  Mastershift Softecu/1(To_GCM) -> Bus Creator2/1
  Bus Creator1/1 -> GCM/2(From CP1)  "SoftECU_Out"
  Trans_Plant/2(ActGear) -> Bus Creator2/2
  Bus Creator2/1 -> Bus Creator1/2  "Trans_CAN_Out"
  GCM/1(CAN Out) -> CAN_Transmit/1(To_CAN)
  GCM/2(To SoftECU) -> Mastershift Softecu/1(From GCM), CP1 SoftEcu/1(From GCM)
  Mastershift Softecu/2(Actuator_Cmds) -> Terminator/1
  connections:
  Trans_Plant/LConn1 -- Clutch_Plant/RConn1
  Shaft/RConn1 -- Clutch_Plant/LConn1
  Trans_Plant/RConn1 -- Trans Output Shaft/RConn1

== system EcoSIM3_P2_C2/Powertrain/Electric Motor  ==
  note: Electric Motor
  " Component Model" : Subsystem
  EM_Receive : Subsystem
  EM_Transmit : Subsystem
  Soft ECU : Subsystem
  To_Plants1 : PMIOPort  Port=1  Side=Right
  To_Battery : Outport
  wires:
  " Component Model"/1(Sensor_Out) -> Soft ECU/2(Sensor_In)
  Soft ECU/2(Actuator_Cmds) -> " Component Model"/1(Actuator_Cmds)
  Soft ECU/1(To_ECUs) -> EM_Transmit/1(To_ECUs)
  EM_Receive/1(From_ECUs) -> Soft ECU/1(From_ECUs)
  " Component Model"/2(To_Battery) -> To_Battery/1
  connections:
  " Component Model"/RConn1 -- To_Plants1/RConn1

== system EcoSIM3_P2_C2/Powertrain/Electrical Storage System ==
  note: ESS
  Charger_Power_In [W] : Inport
  Accessories_Power_In [W] : Inport  Port=2
  EM_Power_In [W] : Inport  Port=3
  BAS_Power_In [W] : Inport  Port=4
  " ESS Model" : Subsystem
  CAN_Revieve : Subsystem
  CAN_Transmit : Subsystem
  Soft ECU : Subsystem
  wires:
  Accessories_Power_In [W]/1 -> " ESS Model"/4(Accessories_Power_In [W])
  " ESS Model"/1(Sensor_Out) -> Soft ECU/2(Sensor_In)
  EM_Power_In [W]/1 -> " ESS Model"/3(EM_Power_In [W])
  Soft ECU/2(Actuator_Cmds) -> " ESS Model"/1(Actuator_Cmds)
  Soft ECU/1(To ECUs) -> CAN_Transmit/1(To_CAN)
  CAN_Revieve/1(From_CAN) -> Soft ECU/1(CAN_In)
  BAS_Power_In [W]/1 -> " ESS Model"/5(BAS_Power_In [W])
  Charger_Power_In [W]/1 -> " ESS Model"/2(Charger_Power_In [W])

== system EcoSIM3_P2_C2/Powertrain/Engine ==
  note: Engine
  " Component Model" : Subsystem
  ICE_Receive : Subsystem
  ICE_Transmit : Subsystem
  Soft ECU : Subsystem
  ICE Output Shaft : PMIOPort  Tag=PMCPort  Port=1  Side=Right
  Fuel_Consumption : Outport
  wires:
  " Component Model"/1(Sensor_Out) -> Soft ECU/2(Sensor_In)
  Soft ECU/2(Actuator_Cmds) -> " Component Model"/1(Actuator_Cmds)
  Soft ECU/1(ICE_Out) -> ICE_Transmit/1(To_ECUs)
  ICE_Receive/1(From_ECUs) -> Soft ECU/1(ICE_In)
  " Component Model"/2(Fuel_Consumption) -> Fuel_Consumption/1
  connections:
  " Component Model"/RConn1 -- ICE Output Shaft/RConn1

== system EcoSIM3_P2_C2/Powertrain/Fuel Tank ==
  note: FUEL TANK
  note: This needs to be beta actuator position
  ICE_m_f_dot [kg/s] : Inport
  Add : Sum  Inputs=+-
  Bus Creator1 : BusCreator  Inputs=2
  Divide : Product  Inputs=/*
  Fuel Density : Constant  Value=Plants.ICE.Mdl.Plant.fuel_property.E85_den
  Fuel Density1 : Constant  Value=Plants.Fuel_Tank.Fuel_Cap_Init
  Gain1 : Gain  Gain=1/1000
  Integrator : Integrator
  Terminator : Terminator
  wires:
  Integrator/1 -> Divide/2
  Fuel Density/1 -> Gain1/1
  Divide/1 -> Bus Creator1/2, Add/2  "Fuel_V_f_used_L"
  ICE_m_f_dot [kg/s]/1 -> Integrator/1
  Add/1 -> Bus Creator1/1  "Fuel_Volume_Left_L"
  Bus Creator1/1 -> Terminator/1  "Fuel_Tank_Signals"
  Fuel Density1/1 -> Add/1
  Gain1/1 -> Divide/1

== system EcoSIM3_P2_C2/Powertrain/Mechanical Coupler ==
  note: MECHANICAL COUPLER
  Inertia2 : fl_lib/Mechanical/Rotational Elements/Inertia  inertia=0.01 kg*m^2  w_specify=off  w_priority=High  w=0 rad/s  t_specify=off  t_priority=High  t=0 N*m
  Sensors : Subsystem
  Simple Gear : sdl_lib/Gears/Simple Gear  ratio=Plants.Mech_Coupler.EM_GR  rotation_direction=1  friction_model=2  T_noload=0.1 N*m  T_nom=5 N*m  efficiency_nom=0.8  efficiency=Plants.Mech_Coupler.EM_Eff  mu_visc=[ 0 0 ] N*m/(rad/s)  w_thr=0.01 rad/s
  EM Output Shaft : PMIOPort  Tag=PMCPort  Port=1  Side=Left
  Trans Output Shaft : PMIOPort  Tag=PMCPort  Port=2  Side=Left
  MC_Coupler_Out : PMIOPort  Tag=PMCPort  Port=3  Side=Right
  connections:
  EM Output Shaft/RConn1 -- Simple Gear/LConn1
  Sensors/RConn1 -- MC_Coupler_Out/RConn1
  Sensors/LConn1 -- Inertia2/LConn1 -- Trans Output Shaft/RConn1 -- Simple Gear/RConn1

== system EcoSIM3_P2_C2/Powertrain/Soft_ECUs_IO ==
  note: 1) Add Subsystem or Model blocks as valid variant choices.
      | 2) You cannot connect blocks at this level. At simulation, connectivity is automatically
      | determined, based on the active variant and port name matching.
  From_Goto : Subsystem  VariantControl=Sim_type == 1
  VNT Kvaser : Subsystem  VariantControl=Sim_type == 3
  VNT Vector : Subsystem  VariantControl=Sim_type == 2

== system EcoSIM3_P2_C2/Powertrain/Vehicle Dynamics ==
  note: Velocity of the vehicle in m/s
  note: VEHICLE DYNAMICS
  note: Negative Torque from brakes
  Beta : Inport
  " Front Right Tire" : sdl_lib/Tires & Vehicles/Tire (Magic Formula)  parameterization=1  F_z1=Plants.Front_wh.Rated_Vertical_Load N  F_x1=Plants.Front_wh.Rated_Peak_Long_Force N  kappa1=Plants.Front_wh.Tire.Slip_At_Peak_Force  B_m=10  C_m=1.9  D_m=1  E_m=0.97  fz0=4e+3 N  p_Cx=1.685  p_Dx=[ 1.21 -0.037 ]  p_Ex=[ 0.344 0.095 -0.02 0 ]  p_Kx=[ 21.51 -0.163 0.245 ]  p_Hx=[ -0.002 0.002 ]  p_Vx=[ 0 0 ]  v_tr_thr=Plants.Front_wh.Tire.Slip_Calculation_Velocity_Threshold m/s  r_e=Plants.Front_wh.Tire.rollrad m  model_compliance=0  stiffness=1e+6 N/m  damping=1000 N/(m/s)  model_inertia=1  inertia=Plants.Front_wh.Wheel_Inertia kg*m^2  initial_velocity=0 rpm  model_resistance=1  resistance_model=1  coeff=Plants.Front_wh.Tire.Constant_coeff  p_tire=250e3 Pa  alpha=-0.003  beta=0.97  coeff_a=84e-4  coeff_b=6.2e-4 s/m  coeff_c=1.6e-4 s^2/m^2  v_thr=Plants.Front_wh.Tire.Velocity_threshold m/s
  1-D Lookup Table : Lookup_n-D  NumberOfTableDimensions=1  BreakpointsForDimension1=Plants.Front_br.Brake_Beta_Cmd  Table=Plants.Front_br.Brake_Friction_Map  InternalRulePriority=Speed  RndMeth=Simplest  InputSameDT=on
  Double-Shoe Brake1 : sdl_lib/Brakes & Detents/Rotational/Double-Shoe Brake  r_drum=Plants.Front_br.Drum_radius mm  r_act=Plants.Front_br.Actuator_location mm  r_pin=Plants.Front_br.Pin_location_rad mm  theta_pin=Plants.Front_br.Pin_location_ang deg  theta_0=Plants.Front_br.Shoe_begin_ang deg  theta_shoe=Plants.Front_br.Shoe_span deg  mu_visc=Plants.Front_br.Viscous_fric_coeff N*m/(rad/s)  mu=Plants.Front_br.Contact_fric_coeff  w_thr=Plants.Front_br.Angular_vel_threshold rad/s
  Double-Shoe Brake2 : sdl_lib/Brakes & Detents/Rotational/Double-Shoe Brake  r_drum=Plants.Rear_br.Drum_radius mm  r_act=Plants.Rear_br.Actuator_location mm  r_pin=Plants.Rear_br.Pin_location_rad mm  theta_pin=Plants.Rear_br.Pin_location_ang deg  theta_0=Plants.Rear_br.Shoe_begin_ang deg  theta_shoe=Plants.Rear_br.Shoe_span deg  mu_visc=Plants.Rear_br.Viscous_fric_coeff N*m/(rad/s)  mu=Plants.Rear_br.Contact_fric_coeff  w_thr=Plants.Rear_br.Angular_vel_threshold rad/s
  Double-Shoe Brake3 : sdl_lib/Brakes & Detents/Rotational/Double-Shoe Brake  r_drum=Plants.Front_br.Drum_radius mm  r_act=Plants.Front_br.Actuator_location mm  r_pin=Plants.Front_br.Pin_location_rad mm  theta_pin=Plants.Front_br.Pin_location_ang deg  theta_0=Plants.Front_br.Shoe_begin_ang deg  theta_shoe=Plants.Front_br.Shoe_span deg  mu_visc=Plants.Front_br.Viscous_fric_coeff N*m/(rad/s)  mu=Plants.Front_br.Contact_fric_coeff  w_thr=Plants.Front_br.Angular_vel_threshold rad/s
  Double-Shoe Brake4 : sdl_lib/Brakes & Detents/Rotational/Double-Shoe Brake  r_drum=Plants.Rear_br.Drum_radius mm  r_act=Plants.Rear_br.Actuator_location mm  r_pin=Plants.Rear_br.Pin_location_rad mm  theta_pin=Plants.Rear_br.Pin_location_ang deg  theta_0=Plants.Rear_br.Shoe_begin_ang deg  theta_shoe=Plants.Rear_br.Shoe_span deg  mu_visc=Plants.Rear_br.Viscous_fric_coeff N*m/(rad/s)  mu=Plants.Rear_br.Contact_fric_coeff  w_thr=Plants.Rear_br.Angular_vel_threshold rad/s
  Front Brake Bias : fl_lib/Physical Signals/Functions/PS Gain  gain=Plants.Front_br.brake_F_propor
  Front Left Tire : sdl_lib/Tires & Vehicles/Tire (Magic Formula)  parameterization=1  F_z1=Plants.Front_wh.Rated_Vertical_Load N  F_x1=Plants.Front_wh.Rated_Peak_Long_Force N  kappa1=Plants.Front_wh.Tire.Slip_At_Peak_Force  B_m=10  C_m=1.9  D_m=1  E_m=0.97  fz0=4e+3 N  p_Cx=1.685  p_Dx=[ 1.21 -0.037 ]  p_Ex=[ 0.344 0.095 -0.02 0 ]  p_Kx=[ 21.51 -0.163 0.245 ]  p_Hx=[ -0.002 0.002 ]  p_Vx=[ 0 0 ]  v_tr_thr=Plants.Front_wh.Tire.Slip_Calculation_Velocity_Threshold m/s  r_e=Plants.Front_wh.Tire.rollrad m  model_compliance=0  stiffness=1e+6 N/m  damping=1000 N/(m/s)  model_inertia=1  inertia=Plants.Front_wh.Wheel_Inertia kg*m^2  initial_velocity=0 rpm  model_resistance=1  resistance_model=1  coeff=Plants.Front_wh.Tire.Constant_coeff  p_tire=250e3 Pa  alpha=-0.003  beta=0.97  coeff_a=84e-4  coeff_b=6.2e-4 s/m  coeff_c=1.6e-4 s^2/m^2  v_thr=Plants.Front_wh.Tire.Velocity_threshold m/s
  PS-Simulink Converter : nesl_utility/PS-Simulink Converter  PhysicalDomain=network_engine_domain  SubClassName=ps_output  LeftPortType=input  RightPortType=output  PseudoPeriodic=off  Frequencies=[]  Unit=1  AffineConversion=off
  PS-Simulink Converter1 : nesl_utility/PS-Simulink Converter  PhysicalDomain=network_engine_domain  SubClassName=ps_output  LeftPortType=input  RightPortType=output  PseudoPeriodic=off  Frequencies=[]  Unit=1  AffineConversion=off
  Rear Differential : sdl_lib/Gears/Differential  driveshaft_location=2  cd_ratio=Plants.Rear_Diff.Diff_ratio  friction_model=2  efficiency=Plants.Rear_Diff.Ordinary_efficiencies  mu_visc=Plants.Rear_Diff.damp N*m/(rad/s)  w_thr=Plants.Rear_Diff.Velocity_thresholds rad/s
  Rear Brake Bias : fl_lib/Physical Signals/Functions/PS Gain  gain=Plants.Rear_br.brake_R_propor
  Rear Right Tire : sdl_lib/Tires & Vehicles/Tire (Magic Formula)  parameterization=1  F_z1=Plants.Rear_wh.Rated_Vertical_Load N  F_x1=Plants.Rear_wh.Rated_Peak_Long_Force N  kappa1=Plants.Rear_wh.Tire.Slip_At_Peak_Force  B_m=10  C_m=1.9  D_m=1  E_m=0.97  fz0=4e+3 N  p_Cx=1.685  p_Dx=[ 1.21 -0.037 ]  p_Ex=[ 0.344 0.095 -0.02 0 ]  p_Kx=[ 21.51 -0.163 0.245 ]  p_Hx=[ -0.002 0.002 ]  p_Vx=[ 0 0 ]  v_tr_thr=Plants.Rear_wh.Tire.Slip_Calculation_Velocity_Threshold m/s  r_e=Plants.Rear_wh.Tire.rollrad m  model_compliance=0  stiffness=1e+6 N/m  damping=1000 N/(m/s)  model_inertia=1  inertia=Plants.Rear_wh.Wheel_Inertia kg*m^2  initial_velocity=0 rpm  model_resistance=1  resistance_model=1  coeff=Plants.Rear_wh.Tire.Constant_coeff  p_tire=250e3 Pa  alpha=-0.003  beta=0.97  coeff_a=84e-4  coeff_b=6.2e-4 s/m  coeff_c=1.6e-4 s^2/m^2  v_thr=Plants.Rear_wh.Tire.Velocity_threshold m/s
  Rear Right Tires : sdl_lib/Tires & Vehicles/Tire (Magic Formula)  parameterization=1  F_z1=Plants.Rear_wh.Rated_Vertical_Load N  F_x1=Plants.Rear_wh.Rated_Peak_Long_Force N  kappa1=Plants.Rear_wh.Tire.Slip_At_Peak_Force  B_m=10  C_m=1.9  D_m=1  E_m=0.97  fz0=4e+3 N  p_Cx=1.685  p_Dx=[ 1.21 -0.037 ]  p_Ex=[ 0.344 0.095 -0.02 0 ]  p_Kx=[ 21.51 -0.163 0.245 ]  p_Hx=[ -0.002 0.002 ]  p_Vx=[ 0 0 ]  v_tr_thr=Plants.Rear_wh.Tire.Slip_Calculation_Velocity_Threshold m/s  r_e=Plants.Rear_wh.Tire.rollrad m  model_compliance=0  stiffness=1e+6 N/m  damping=1000 N/(m/s)  model_inertia=1  inertia=Plants.Rear_wh.Wheel_Inertia kg*m^2  initial_velocity=0 rpm  model_resistance=1  resistance_model=1  coeff=Plants.Rear_wh.Tire.Constant_coeff  p_tire=250e3 Pa  alpha=-0.003  beta=0.97  coeff_a=84e-4  coeff_b=6.2e-4 s/m  coeff_c=1.6e-4 s^2/m^2  v_thr=Plants.Rear_wh.Tire.Velocity_threshold m/s
  Road Grade : fl_lib/Physical Signals/Sources/PS Constant  constant=0
  Scope1 : Scope  Commented=on  NumInputPorts=2
      settings: TimeRange=0.05746676406135975  YMin=-0.001119~-0.000858  YMax=-0.00111~-0.00084  SaveName=ScopeData11
  Sensor : Subsystem
  Simulink-PS Converter1 : nesl_utility/Simulink-PS Converter  PhysicalDomain=network_engine_domain  SubClassName=ps_input  LeftPortType=input  RightPortType=output  PseudoPeriodic=off  Frequencies=[]  NoiseDistribution=none  NoiseParameters=[]  Unit=N  AffineConversion=off  InputFiltering=off  SimscapeFilterOrder=1  InputFilterTimeConstant=0.001  UdotUserProvided=1
  Subsystem : Subsystem
  Vehicle Body : sdl_lib/Tires & Vehicles/Vehicle Body  mass=Veh_Dynamics.Body.Mass kg  n_w=2  x_f=Veh_Dynamics.Body.Distance_CG_FrontAxle m  x_r=Veh_Dynamics.Body.Distance_CG_RearAxle m  y_c=Veh_Dynamics.Body.Distance_CG_Ground m  area=Veh_Dynamics.Body.Frontal_Area m^2  Cd=Veh_Dynamics.Body.Aero_Drag_Coeff  v0=0 m/s  g=9.81 m/s^2  rho=1.18 kg/m^3
  Wind velocity : fl_lib/Physical Signals/Sources/PS Constant  constant=0
  MC_Coupler_Out : PMIOPort  Tag=PMCPort  Port=1  Side=Left
  Vehicle_Speed [m/s] : Outport
  wires:
  PS-Simulink Converter/1 -> Scope1/1  "LF_Wheel_Slip"
  PS-Simulink Converter1/1 -> Scope1/2  "LR_Wheel_Slip"
  Beta/1 -> 1-D Lookup Table/1
  1-D Lookup Table/1 -> Simulink-PS Converter1/1
  Sensor/1(Sensor_Out) -> Vehicle_Speed [m/s]/1
  connections:
  " Front Right Tire"/LConn1 -- Vehicle Body/RConn2 -- Front Left Tire/LConn1
  Rear Right Tire/LConn1 -- Vehicle Body/RConn1 -- Rear Right Tires/LConn1
  Rear Right Tires/LConn2 -- Sensor/RConn1 -- Rear Differential/RConn2 -- Double-Shoe Brake2/LConn2
  Rear Right Tire/LConn2 -- Double-Shoe Brake4/LConn2 -- Sensor/RConn2 -- Rear Differential/RConn1
  " Front Right Tire"/RConn2 -- Front Left Tire/RConn2 -- Subsystem/RConn1 -- Rear Right Tire/RConn2 -- Rear Right Tires/RConn2
  Rear Brake Bias/LConn1 -- Simulink-PS Converter1/RConn1 -- Front Brake Bias/LConn1
  Double-Shoe Brake3/LConn1 -- Double-Shoe Brake1/LConn1 -- Front Brake Bias/RConn1
  Front Left Tire/LConn2 -- Sensor/LConn3 -- " Front Right Tire"/LConn2 -- Sensor/LConn2 -- Double-Shoe Brake1/LConn2 -- Double-Shoe Brake3/LConn2
  Double-Shoe Brake2/LConn1 -- Rear Brake Bias/RConn1 -- Double-Shoe Brake4/LConn1
  Subsystem/LConn1 -- Vehicle Body/LConn1
  Road Grade/RConn1 -- Vehicle Body/RConn3
  PS-Simulink Converter1/LConn1 -- Rear Right Tires/RConn1
  PS-Simulink Converter/LConn1 -- " Front Right Tire"/RConn1
  Vehicle Body/LConn2 -- Sensor/LConn1
  MC_Coupler_Out/RConn1 -- Rear Differential/LConn1
  Vehicle Body/LConn3 -- Wind velocity/RConn1

== system EcoSIM3_P2_C2/RTI Data/RTI Data Store ==
  RTI Data Store : Subsystem  mask(RTI_DATA_STORE){}
      mask help:
      | RTI Data Store Block. This block is used by RTI to store internal model dependent data. Deleting this block will result in data loss.
      |
      | NEVER DELETE, COPY, OR MODIFY THIS BLOCK!
      mask Help:
      | RTI Data Store Block. This block is used by RTI to store internal model dependent data. Deleting this block will result in data loss.
      | 
      | NEVER DELETE, COPY, OR MODIFY THIS BLOCK!
      mask Display: text(0.5, 0.5, ' ', 'HorizontalAlignment', 'center');
